simulink model "obiekt_regulacji"  (R2019b)
settings: Solver=VariableStepAuto  StartTime=0.0  StopTime=40  RelTol=1e-3
values from neighbouring files (symbols this model uses):
  k = str2num(answer{1,1})    [index.m]
  T0 = str2num(answer{7,1})    [index.m]
  T1 = str2num(answer{2,1})    [index.m]
  T2 = str2num(answer{3,1})    [index.m]
  T3 = str2num(answer{4,1})    [index.m]
  T4 = str2num(answer{5,1})    [index.m]
  T5 = str2num(answer{6,1})    [index.m]
settings Model: Creator=01129847  LastModifiedBy=01129847
settings DataIOCC: SaveOutput=off  SaveTime=off

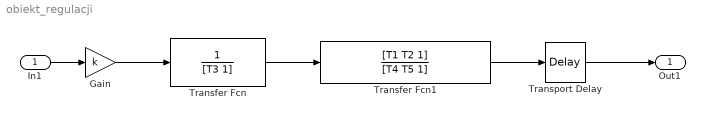
== system obiekt_regulacji ==
  In1 : Inport  OutDataTypeStr=double  PortDimensions=1  SampleTime=[0,1]
  Gain : Gain  Gain=k
  Transfer Fcn : TransferFcn  Denominator=[T3 1]
  Transfer Fcn1 : TransferFcn  Numerator=[T1 T2 1]  Denominator=[T4 T5 1]
  Transport Delay : TransportDelay  DelayTime=T0
  Out1 : Outport  OutDataTypeStr=double  PortDimensions=1  SampleTime=0
  wires:
  In1/1 -> Gain/1
  Gain/1 -> Transfer Fcn/1
  Transfer Fcn1/1 -> Transport Delay/1
  Transfer Fcn/1 -> Transfer Fcn1/1
  Transport Delay/1 -> Out1/1
